simulink model "Quater_car_model_Tire1"  (R2023b)
settings: Solver=ode4  StartTime=0.0  StopTime=10.0  FixedStep=0.00001  RelTol=1e-3
undefined symbols (not defined in the file): B1, C1, Cx, D1, D_brake, E1, Ip, Kx, m1, m2, mu, N, R1, R2, reff, Rm, Sh, Sv, Vo
libraries: slpidlib x1
settings Model: Creator=Santhosh  LastModifiedBy=Santhosh

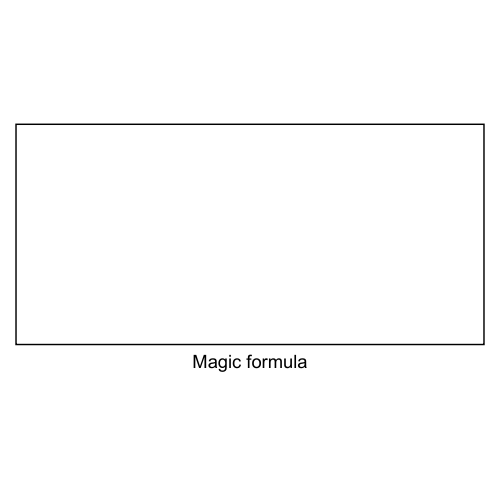
[thumbnail: Simulink's stored preview of the top-level diagram]
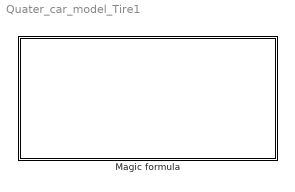
== system Quater_car_model_Tire1 ==
  Magic formula : Subsystem

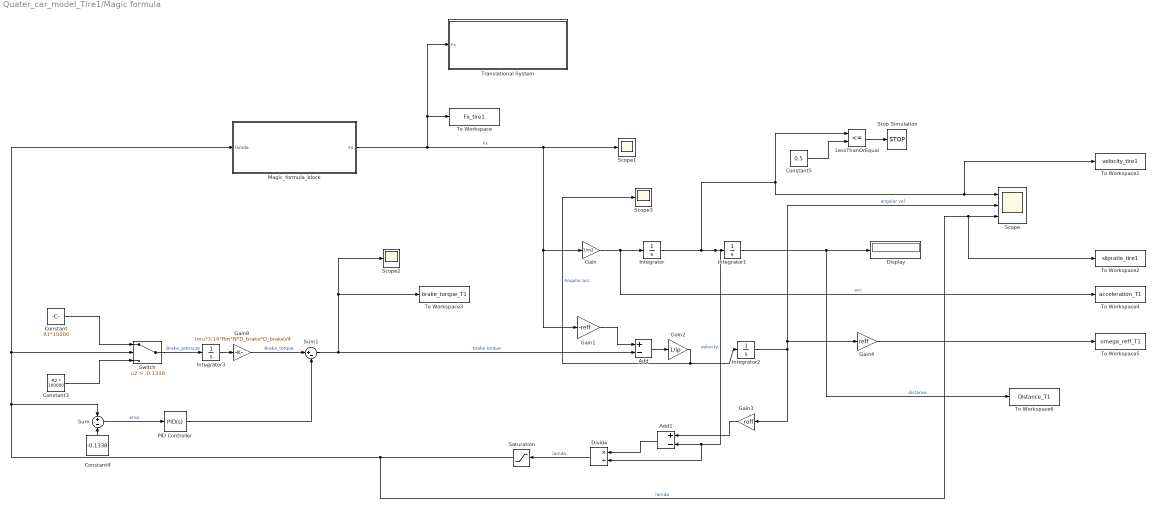
== system Quater_car_model_Tire1/Magic formula ==
  Add : Sum  Inputs=+-
  Add1 : Sum  Inputs=+-
  Constant : Constant  Value=R1*10000
  Constant3 : Constant  Value=-R2 * 100000
  Constant4 : Constant  Value=-0.1338
  Constant5 : Constant  Value=0.5
  Display : Display
  Divide : Product  Inputs=*/
  Gain : Gain  Gain=1/m2
  Gain1 : Gain  Gain=-reff
  Gain2 : Gain  Gain=1/Ip
  Gain3 : Gain  Gain=reff
  Gain4 : Gain  Gain=reff
  Gain8 : Gain  Gain=(mu*3.14*Rm*N*D_brake*D_brake)/4
  Integrator : Integrator  InitialCondition=Vo
  Integrator1 : Integrator
  Integrator2 : Integrator  InitialCondition=Vo/reff
  Integrator3 : Integrator
  LessThanOrEqual : RelationalOperator  Operator=<=  OutDataTypeStr=boolean  RndMeth=Simplest  InputSameDT=off
  Magic_formula_block : Subsystem
  PID Controller : slpidlib/PID Controller  Controller=PID  Form=Parallel  TimeDomain=Continuous-time  UseExternalTs=off  SampleTime=-1  IntegratorMethod=Forward Euler  FilterMethod=Forward Euler  ControllerParametersSource=internal  P=-251638.942322948  I=-88129068.0592158  UseKiTs=off  D=15.1380068237289  N=3591.92303243582  UseFilter=on  TunerSelectOption=Frequency Response Based  InitialConditionSource=internal  InitialConditionForIntegrator=0  InitialConditionForFilter=0  DifferentiatorICPrevScaledInput=0  ExternalReset=none  TrackingMode=off  Kt=1  LimitOutput=off  SatLimitsSource=internal  UpperSaturationLimit=inf  LowerSaturationLimit=-inf  LinearizeAsGain=on  AntiWindupMode=none  Kb=1  LimitIntegrator=off  UpperIntegratorSaturationLimit=inf  LowerIntegratorSaturationLimit=-inf  POutMin=[]  POutMax=[]  IOutMin=[]  IOutMax=[]  DOutMin=[]  DOutMax=[]  NOutMin=[]  NOutMax=[]  SumOutMin=[]  SumOutMax=[]  SaturationOutMin=[]  SaturationOutMax=[]  PParamMin=[]  PParamMax=[]  IParamMin=[]  IParamMax=[]  DParamMin=[]  DParamMax=[]  NParamMin=[]  NParamMax=[]  KbParamMin=[]  KbParamMax=[]  KtParamMin=[]  KtParamMax=[]  KbOutMin=[]  KbOutMax=[]  KtOutMin=[]  KtOutMax=[]  IntegratorOutMin=[]  IntegratorOutMax=[]  FilterOutMin=[]  FilterOutMax=[]  SumI1OutMin=[]  SumI1OutMax=[]  SumI2OutMin=[]  SumI2OutMax=[]  SumI3OutMin=[]  SumI3OutMax=[]  SumI4OutMin=[]  SumI4OutMax=[]  SumDOutMin=[]  SumDOutMax=[]  DifferentiatorOutMin=[]  DifferentiatorOutMax=[]  FilterDiffOutCoefMin=[]  FilterDiffOutCoefMax=[]  ReciprocalOutMin=[]  ReciprocalOutMax=[]  SumDenOutMin=[]  SumDenOutMax=[]  SumNumOutMin=[]  SumNumOutMax=[]  DivideOutMin=[]  DivideOutMax=[]  UdiffTsProdOutMin=[]  UdiffTsProdOutMax=[]  NTsProdOutMin=[]  NTsProdOutMax=[]  UintegralTsProdOutMin=[]  UintegralTsProdOutMax=[]  UngainTsProdOutMin=[]  UngainTsProdOutMax=[]  ClampingZeroOutDataTypeStr=Inherit: Inherit via back propagation  ClampingZeroOutMin=[]  ClampingZeroOutMax=[]  FilterDenConstantOutDataTypeStr=Inherit: Inherit via back propagation  FilterDenConstantOutMin=[]  FilterDenConstantOutMax=[]  PCopyOutDataTypeStr=Inherit: Inherit via back propagation  PCopyOutMin=[]  PCopyOutMax=[]  NCopyOutDataTypeStr=Inherit: Inherit via back propagation  NCopyOutMin=[]  NCopyOutMax=[]  IntegratorContinuousStateAttributes=''  IntegratorStateMustResolveToSignalObject=off  IntegratorRTWStateStorageClass=Auto  FilterContinuousStateAttributes=''  FilterStateMustResolveToSignalObject=off  FilterRTWStateStorageClass=Auto  ParallelPVariant=InternalParameters  IdealPVariant=Disabled  IVariant=InternalParameters  DVariant=InternalParameters  IntegratorVariant=Continuous  SatVariant=Disabled  AWVariant=Passthrough  PCopyVariant=Disabled  TRVariant=Disabled  FdbkBlocksVariant=Forward  IdealPFdbkVariant=Disabled  SatFdbkVariant=Disabled  DerivativeFilterVariant=ContFilter  NVariant=InternalParameters  NCopyVariant=Disabled  FilterICVariant=InternalICsFilter  IntegratorICVariant=InternalICs  ExternalResetVariant=Disabled  TRSumVariant=Passthrough  SumFdbkVariant=Disabled  SumVariant=Sum_PID  TsampFilterVariant=InternalTs  TsampNgainVariant=Passthrough  TsampIntegralVariant=Disabled_SignalSpec  ExternalSaturationOutDataTypeStr=Inherit: Same as second input
  Saturation : Saturate  UpperLimit=1  LowerLimit=-1
  Scope : Scope  NumInputPorts=3
  Scope1 : Scope
  Scope2 : Scope
  Scope3 : Scope
  Stop Simulation : Stop
  Sum : Sum  Inputs=+-
  Sum1 : Sum  Inputs=|+-
  Switch : Switch  Criteria=u2 > Threshold  Threshold=-0.1338  SaturateOnIntegerOverflow=off  InputSameDT=off
  To Workspace : ToWorkspace  VariableName=Fx_tire1  SaveFormat=Timeseries  SampleTime=-1
  To Workspace1 : ToWorkspace  VariableName=velocity_tire1  SaveFormat=Timeseries  SampleTime=-1
  To Workspace2 : ToWorkspace  VariableName=slipratio_tire1  SaveFormat=Timeseries  SampleTime=-1
  To Workspace3 : ToWorkspace  VariableName=brake_torque_T1  SaveFormat=Timeseries  SampleTime=-1
  To Workspace4 : ToWorkspace  VariableName=acceleration_T1  SaveFormat=Timeseries  SampleTime=-1
  To Workspace5 : ToWorkspace  VariableName=omega_reff_T1  SaveFormat=Timeseries  SampleTime=-1
  To Workspace6 : ToWorkspace  VariableName=Distance_T1  SaveFormat=Timeseries  SampleTime=-1
  Translational System : Subsystem
  wires:
  Gain/1 -> To Workspace4/1, Integrator/1  "acc"
  Integrator/1 -> Add1/2, Divide/2, Integrator1/1, LessThanOrEqual/1, To Workspace1/1, Scope/1  "velocity"
  Integrator1/1 -> To Workspace6/1, Display/1  "distance"
  Gain1/1 -> Add/1
  Add/1 -> Gain2/1
  Gain2/1 -> Integrator2/1, Scope3/1  "Angular acc"
  Integrator2/1 -> Scope/2, Gain4/1, Gain3/1  "angular vel"
  Gain3/1 -> Add1/1
  Add1/1 -> Divide/1
  Divide/1 -> Saturation/1  "lamda"
  Saturation/1 -> To Workspace2/1, Scope/3, Magic_formula_block/1(lamda), Switch/2, Sum/1  "lamda"
  Constant/1 -> Switch/1
  Constant3/1 -> Switch/3
  Switch/1 -> Integrator3/1  "Brake_pressure"
  Constant4/1 -> Sum/2
  Sum/1 -> PID Controller/1  "error"
  PID Controller/1 -> Sum1/2
  Gain8/1 -> Sum1/1  "Brake_torque"
  Sum1/1 -> Scope2/1, To Workspace3/1, Add/2  "brake torque"
  Constant5/1 -> LessThanOrEqual/2
  LessThanOrEqual/1 -> Stop Simulation/1
  Magic_formula_block/1(Fx) -> To Workspace/1, Translational System/1(Fx), Scope1/1, Gain1/1, Gain/1  "Fx"
  Gain4/1 -> To Workspace5/1
  Integrator3/1 -> Gain8/1

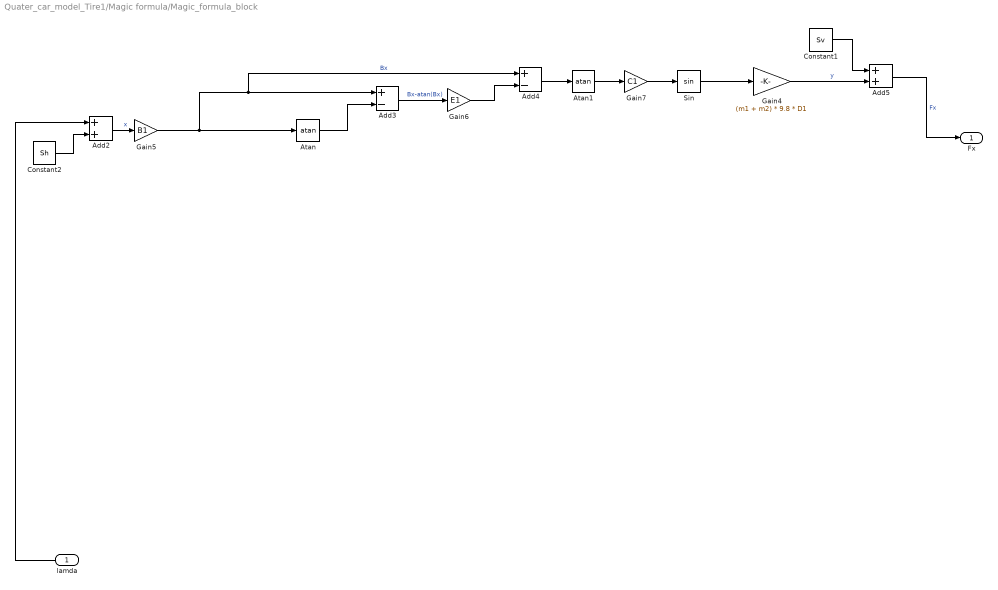
== system Quater_car_model_Tire1/Magic formula/Magic_formula_block ==
  lamda : Inport
  Add2 : Sum
  Add3 : Sum  Inputs=+-
  Add4 : Sum  Inputs=+-
  Add5 : Sum
  Atan : Trigonometry  Operator=atan
  Atan1 : Trigonometry  Operator=atan
  Constant1 : Constant  Value=Sv
  Constant2 : Constant  Value=Sh
  Gain4 : Gain  Gain=(m1 + m2) * 9.8 * D1
  Gain5 : Gain  Gain=B1
  Gain6 : Gain  Gain=E1
  Gain7 : Gain  Gain=C1
  Sin : Trigonometry
  Fx : Outport
  wires:
  Gain5/1 -> Atan/1, Add3/1, Add4/1  "Bx"
  Constant2/1 -> Add2/2
  Add2/1 -> Gain5/1  "x"
  Atan1/1 -> Gain7/1
  Gain4/1 -> Add5/2  "y"
  Add4/1 -> Atan1/1
  Gain7/1 -> Sin/1
  Atan/1 -> Add3/2
  Gain6/1 -> Add4/2
  Constant1/1 -> Add5/1
  Add3/1 -> Gain6/1  "Bx-atan(Bx)"
  Sin/1 -> Gain4/1
  Add5/1 -> Fx/1  "Fx"
  lamda/1 -> Add2/1

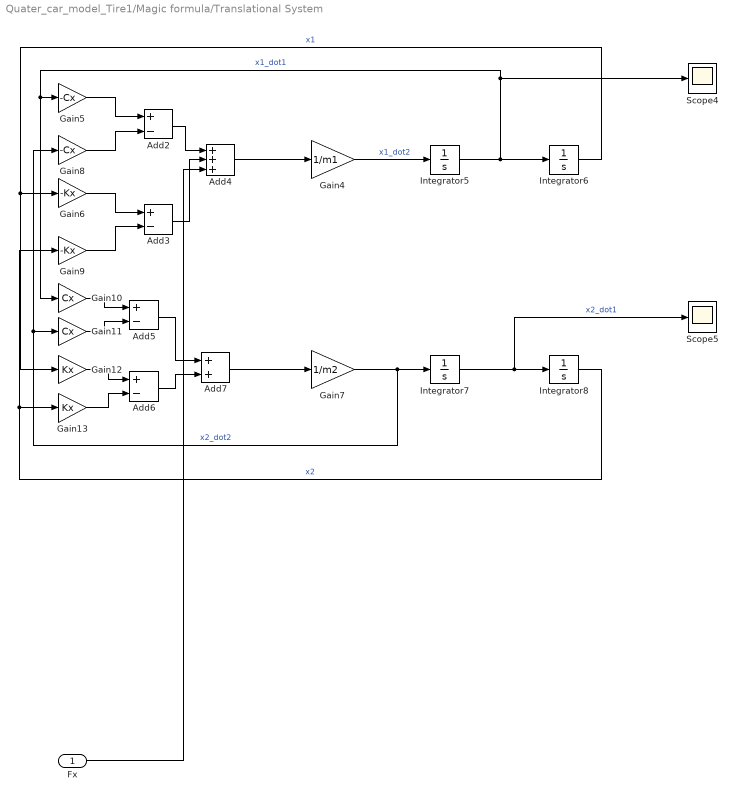
== system Quater_car_model_Tire1/Magic formula/Translational System ==
  Fx : Inport
  Add{2..3,5..6} (4 alike) : Sum  Inputs=+-
  Add4 : Sum  Inputs=+++
  Add7 : Sum
  Gain10 : Gain  Gain=Cx
  Gain11 : Gain  Gain=Cx
  Gain12 : Gain  Gain=Kx
  Gain13 : Gain  Gain=Kx
  Gain4 : Gain  Gain=1/m1
  Gain5 : Gain  Gain=-Cx
  Gain6 : Gain  Gain=-Kx
  Gain7 : Gain  Gain=1/m2
  Gain8 : Gain  Gain=-Cx
  Gain9 : Gain  Gain=-Kx
  Integrator{5..8} (4 alike) : Integrator
  Scope4 : Scope
  Scope5 : Scope
  wires:
  Gain4/1 -> Integrator5/1  "x1_dot2"
  Gain6/1 -> Add3/1
  Add7/1 -> Gain7/1
  Add6/1 -> Add7/2
  Add4/1 -> Gain4/1
  Integrator5/1 -> Scope4/1, Gain10/1, Gain5/1, Integrator6/1  "x1_dot1"
  Integrator7/1 -> Scope5/1, Integrator8/1  "x2_dot1"
  Gain10/1 -> Add5/1
  Integrator8/1 -> Gain13/1, Gain9/1  "x2"
  Gain13/1 -> Add6/2
  Gain8/1 -> Add2/2
  Gain7/1 -> Gain11/1, Gain8/1, Integrator7/1  "x2_dot2"
  Add5/1 -> Add7/1
  Fx/1 -> Add4/3
  Add2/1 -> Add4/1
  Gain5/1 -> Add2/1
  Add3/1 -> Add4/2
  Integrator6/1 -> Gain6/1, Gain12/1  "x1"
  Gain11/1 -> Add5/2
  Gain12/1 -> Add6/1
  Gain9/1 -> Add3/2
